simulink model "simulink_unity"  (R2021a)
settings: Solver=ode1  StartTime=0.0  StopTime=inf  FixedStep=1e-3  RelTol=1e-3
values from neighbouring files (symbols this model uses):
  F_ext = zeros(6,n_q+2)    [simulation_init_unity.m]
  finger_r = Finger('Index', 'RRRR', finger_dimension)    [simulation_init_unity.m]
  Kd = [1;1;1;1]    [simulation_init_unity.m]
  Ks = [100;100;100;100]    [simulation_init_unity.m]
  mdh_ne = mdh_struct_to_matrix(finger_r.mdh_ori, 1)    [simulation_init_unity.m]
  q_init = [0;0;0;0]*pi/180    [simulation_init_unity.m]
  qD_init = [0;0;0;0]*pi/180    [simulation_init_unity.m]
libraries: unity_lib_UDP x1
settings Model: Creator=ge26jow  LastModifiedBy=ge26jow

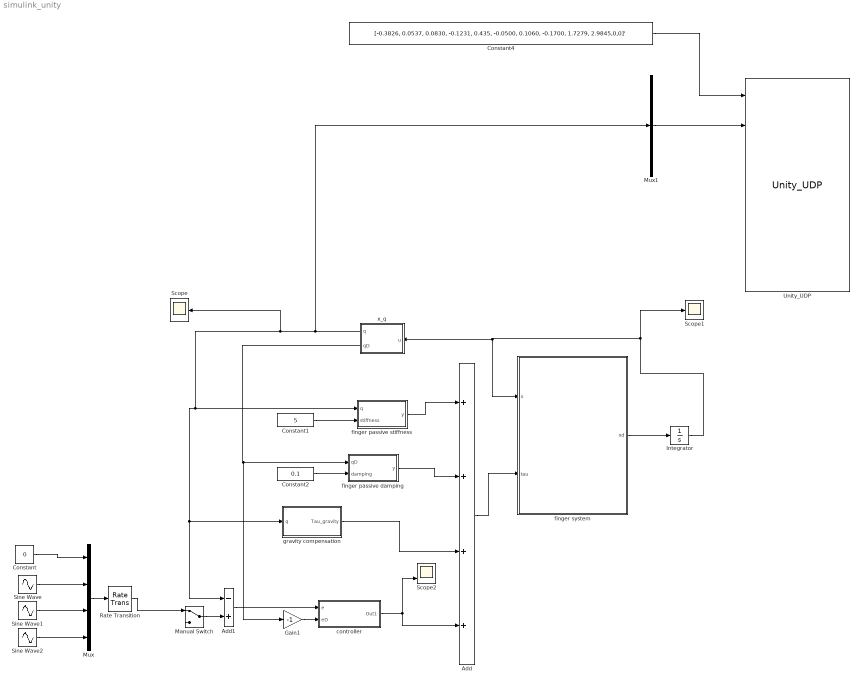
== system simulink_unity ==
  Add : Sum  Inputs=++++
  Add1 : Sum  Inputs=-+
  Constant : Constant  Value=0
  Constant1 : Constant  Value=5
  Constant2 : Constant  Value=0.1
  Constant4 : Constant  Value=[-0.3826, 0.0537, 0.0830, -0.1231, 0.435, -0.0500, 0.1060, -0.1700, 1.7279, 2.9845,0,0]'
  Gain1 : Gain  Gain=-1
  Integrator : Integrator  InitialCondition=[q_init;qD_init]  WrappedStateUpperValue=[pi,pi,pi,pi,1e4,1e4,1e4,1e4]  WrappedStateLowerValue=-[pi,pi,pi,pi,1e4,1e4,1e4,1e4]
  Manual Switch : ManualSwitch
  Mux : Mux
  Mux1 : Mux  Inputs=[6,4,16]
  Rate Transition : RateTransition  OutPortSampleTime=1e-2
  Scope : Scope
  Scope1 : Scope
  Scope2 : Scope  NumInputPorts=2
  Sine Wave : Sin  Amplitude=0.5  Bias=0.5
  Sine Wave1 : Sin  Amplitude=0.5  Bias=0.5
  Sine Wave2 : Sin  Amplitude=0.5  Bias=0.5
  Unity_UDP : unity_lib_UDP/Unity_UDP  IP_port=8051  sampling_time=1e-2
  controller : Subsystem
  finger passive damping : MATLAB Function  TreatAsAtomicUnit=on
  finger passive stiffness : MATLAB Function  TreatAsAtomicUnit=on
  finger system : Subsystem
  gravity compensation : Subsystem
  x_q : MATLAB Function  TreatAsAtomicUnit=on
  wires:
  finger system/1(xd) -> Integrator/1
  x_q/1(q) -> Mux1/2, finger passive stiffness/1(q), Add1/1, gravity compensation/1(q), Scope/1
  Add/1 -> finger system/2(tau)
  finger passive stiffness/1(y) -> Add/1
  finger passive damping/1(y) -> Add/2
  x_q/2(qD) -> Gain1/1, finger passive damping/1(qD)
  Constant1/1 -> finger passive stiffness/2(stiffness)
  Constant2/1 -> finger passive damping/2(damping)
  Add1/1 -> controller/1(e)
  controller/1(Out1) -> Scope2/2, Add/4
  Gain1/1 -> controller/2(eD)
  Integrator/1 -> Scope1/1, finger system/1(x), x_q/1(u)
  Mux1/1 -> Unity_UDP/2
  Sine Wave/1 -> Mux/2
  Constant/1 -> Mux/1
  Sine Wave1/1 -> Mux/3
  Sine Wave2/1 -> Mux/4
  Manual Switch/1 -> Add1/2
  Mux/1 -> Rate Transition/1
  Rate Transition/1 -> Manual Switch/1
  Constant4/1 -> Unity_UDP/1
  gravity compensation/1(Tau_gravity) -> Add/3

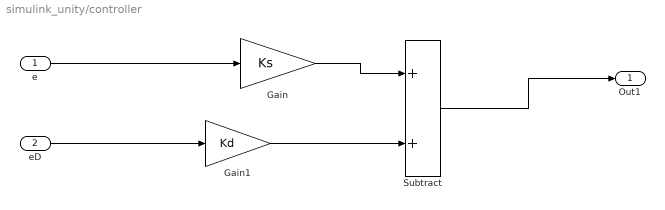
== system simulink_unity/controller ==
  e : Inport
  eD : Inport  Port=2
  Gain : Gain  Gain=Ks
  Gain1 : Gain  Gain=Kd
  Subtract : Sum
  Out1 : Outport
  wires:
  e/1 -> Gain/1
  Gain/1 -> Subtract/1
  eD/1 -> Gain1/1
  Gain1/1 -> Subtract/2
  Subtract/1 -> Out1/1

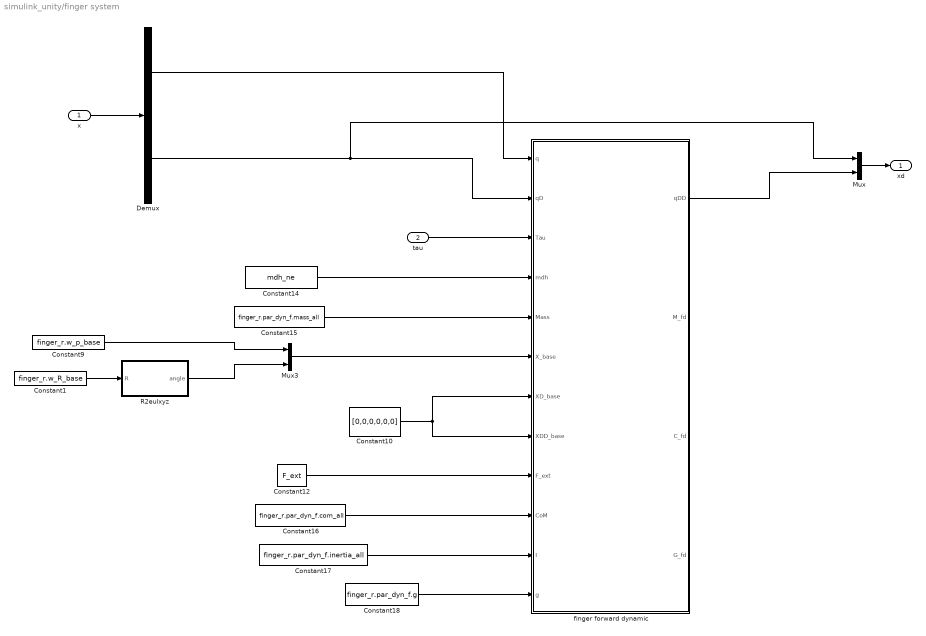
== system simulink_unity/finger system ==
  x : Inport  PortDimensions=8
  tau : Inport  Port=2
  Constant1 : Constant  Value=finger_r.w_R_base
  Constant10 : Constant  Value=[0,0,0,0,0,0]
  Constant12 : Constant  Value=F_ext
  Constant14 : Constant  Value=mdh_ne
  Constant15 : Constant  Value=finger_r.par_dyn_f.mass_all
  Constant16 : Constant  Value=finger_r.par_dyn_f.com_all
  Constant17 : Constant  Value=finger_r.par_dyn_f.inertia_all
  Constant18 : Constant  Value=finger_r.par_dyn_f.g
  Constant9 : Constant  Value=finger_r.w_p_base
  Demux : Demux  Outputs=[4,4]
  Mux : Mux  Inputs=2
  Mux3 : Mux  Inputs=[3,3]
  R2eulxyz : MATLAB Function  TreatAsAtomicUnit=on
  finger forward dynamic : MATLAB Function  TreatAsAtomicUnit=on
  xd : Outport
  wires:
  Constant18/1 -> finger forward dynamic/12(g)
  tau/1 -> finger forward dynamic/3(Tau)
  Constant17/1 -> finger forward dynamic/11(I)
  finger forward dynamic/1(qDD) -> Mux/2
  Constant10/1 -> finger forward dynamic/7(XD_base), finger forward dynamic/8(XDD_base)
  Demux/2 -> Mux/1, finger forward dynamic/2(qD)
  Mux3/1 -> finger forward dynamic/6(X_base)
  Constant14/1 -> finger forward dynamic/4(mdh)
  Demux/1 -> finger forward dynamic/1(q)
  Constant12/1 -> finger forward dynamic/9(F_ext)
  Constant15/1 -> finger forward dynamic/5(Mass)
  Constant16/1 -> finger forward dynamic/10(CoM)
  Mux/1 -> xd/1
  x/1 -> Demux/1
  Constant1/1 -> R2eulxyz/1(R)
  R2eulxyz/1(angle) -> Mux3/2
  Constant9/1 -> Mux3/1

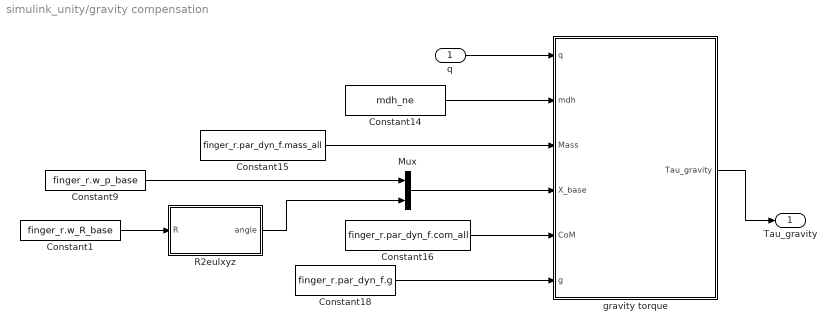
== system simulink_unity/gravity compensation ==
  q : Inport
  Constant1 : Constant  Value=finger_r.w_R_base
  Constant14 : Constant  Value=mdh_ne
  Constant15 : Constant  Value=finger_r.par_dyn_f.mass_all
  Constant16 : Constant  Value=finger_r.par_dyn_f.com_all
  Constant18 : Constant  Value=finger_r.par_dyn_f.g
  Constant9 : Constant  Value=finger_r.w_p_base
  Mux : Mux  Inputs=[3,3]
  R2eulxyz : MATLAB Function  TreatAsAtomicUnit=on
  "gravity torque " : MATLAB Function  TreatAsAtomicUnit=on
  Tau_gravity : Outport
  wires:
  Constant14/1 -> "gravity torque "/2(mdh)
  Constant16/1 -> "gravity torque "/5(CoM)
  Mux/1 -> "gravity torque "/4(X_base)
  Constant18/1 -> "gravity torque "/6(g)
  Constant15/1 -> "gravity torque "/3(Mass)
  "gravity torque "/1(Tau_gravity) -> Tau_gravity/1
  q/1 -> "gravity torque "/1(q)
  Constant1/1 -> R2eulxyz/1(R)
  Constant9/1 -> Mux/1
  R2eulxyz/1(angle) -> Mux/2

== matlab function simulink_unity/x_q ==
  data: u input; q output; qD output
function [q,qD] = fcn(u)

q = u(1:4);
qD = u(5:8);

== matlab function simulink_unity/finger system/finger forward dynamic ==
  data: q input; qDD output; qD input; Tau input; mdh input; Mass input; X_base input; XD_base input; XDD_base input; F_ext input; CoM input; I input; g input; M_fd output; C_fd output; G_fd output
% recursive Newton-Euler method to compute inverse dynamic with mdh
% parameters
% Input:
%     q,qD:             [n_qx1] joint states
%     Tau               [n_q] joint torque
%     mdh:              [n_q+1x4] in sequence of [alpha,a,theta,d] To be
%                       noted that the theta should exclude from mdh parameters 
%     Mass:             [n_q+1] mass vector. the first mass is the base 
%     X_base:           [6x1] eulerxyz
%     XD_base:          [6x1] translational and angular velocity
%     F_ext:            [6x1] force/moment that exerted by the environment to the endeffector frame. 
%     CoM:              [3xn_q+1] in local frame; last column is endeffector
%     I:                [6xn_q+1] in local frame with respect to center of mass. in sequence of [xx yy zz yz xz xy]
%     g:                [3x1] gravity term
% 
% Output:
%     qDD:              [n_qx1] joint acceleration 
%     M_fd:             [n_qxn_q] Mass matrix 
%     C_fd:             [n_q] velocity-dependent torque 
%     G_fd:             [n_q] gravity torque  

function [qDD,M_fd,C_fd,G_fd] = fordyn_ne_mdh(q,qD,Tau,mdh, Mass, X_base, XD_base,XDD_base, F_ext, CoM, I, g)
coder.extrinsic('invdyn_ne_mdh_mex');

n_q = length(q);
% assert(n_q == length(qD)&&n_q == length(Tau),'fordyn_ne_mdh: dimension error!');

mex = 1;


M_fd = zeros(n_q,n_q);
G_fd = zeros(n_q,1);
C_fd = zeros(n_q,1);

% gravity term
if mex
    G_fd = invdyn_ne_mdh_mex(q,zeros(n_q,1),zeros(n_q,1),mdh, Mass,...
        X_base, XD_base, XDD_base, zeros(6,1), CoM, I, g);
else
    G_fd = invdyn_ne_mdh(q,zeros(n_q,1),zeros(n_q,1),mdh, Mass,...
        X_base, XD_base, XDD_base, zeros(6,1), CoM, I, g);
end
% C term
if mex
    C_fd = invdyn_ne_mdh_mex(q,qD,zeros(n_q,1),mdh, Mass,...
        X_base, XD_base, XDD_base, zeros(6,1), CoM, I, g);
else
    C_fd = invdyn_ne_mdh(q,qD,zeros(n_q,1),mdh, Mass,...
             X_base, XD_base, XDD_base, zeros(6,1), CoM, I, g);
end
C_fd = C_fd - G_fd;

% M term
M_fd = zeros(n_q,n_q);

for i = 1:n_q
    qDD_M = zeros(n_q,1);
    qDD_M(i) = 1;
    if mex
        M_fd(:,i) = invdyn_ne_mdh_mex(q,zeros(n_q,1),qDD_M,mdh, Mass,...
            X_base, XD_base, XDD_base, zeros(6,1), CoM, I, g);
    else
        M_fd(:,i) = invdyn_ne_mdh(q,zeros(n_q,1),qDD_M,mdh, Mass,...
            X_base, XD_base, XDD_base, zeros(6,1), CoM, I, g);
    end
    M_fd(:,i) = M_fd(:,i) - G_fd;
end

% use Jacobian_geom_mdh.m to calculate geometric Jacobian
w_R_b = euler2R_XYZ(X_base(4:6));
b_J = Jacobian_geom_mdh(mdh,q);
J_ne = blkdiag(w_R_b,w_R_b)*b_J;
tau_ext = zeros(n_q,1);
for i = 1:n_q+1
    mdh_i = mdh(1:i,:);
    q_i = q(1:min(i,n_q));
    b_J_i = zeros(6,n_q);
    b_J_i(:,1:min(i,n_q)) =  Jacobian_geom_mdh(mdh_i,q_i);
    J_ne_i= blkdiag(w_R_b,w_R_b)*b_J_i;
    tau_i = J_ne_i'*F_ext(:,i+1);
    tau_ext = tau_ext + tau_i;
end


qDD = (M_fd)\(Tau + tau_ext - G_fd - C_fd);


end

== matlab function simulink_unity/finger passive stiffness ==
  data: q input; y output; stiffness input
function y = fcn(q,stiffness)

y = -stiffness.*q;

== matlab function simulink_unity/finger passive damping ==
  data: qD input; y output; damping input
function y = fcn(qD,damping)

y = -damping.*qD;

== matlab function simulink_unity/gravity compensation/gravity torque  ==
  data: q input; Tau_gravity output; mdh input; Mass input; X_base input; CoM input; g input
function Tau_gravity = fcn(q,mdh, Mass, X_base, CoM, g)

Tau_gravity = invdyn_ne_mdh_all_fext_gravity(q,mdh, Mass, X_base, CoM, g);

== matlab function simulink_unity/gravity compensation/R2eulxyz ==
  data: R input; angle output
function angle = fcn(R)

angle = R2euler_XYZ(R);

== matlab function simulink_unity/finger system/R2eulxyz ==
  data: R input; angle output
function angle = fcn(R)

angle = R2euler_XYZ(R);
